simulink library "SLUGS_Library"  (Simulink 6.6)
values from neighbouring files (symbols this model uses):
  T = 0.01    [initGPS.m]    (also in mcuInit.m)
undefined symbols (not defined in the file or in its folder): apSampleTime, bankCommandLimit, daLimit, deLimit, DiscIntNeverNeededParam, drLimit, dtLimit, gaind, getWP, heightErrorLimit, mass, Ndelay, param, pitchCommandLimit, pitchErrorLimit, polesd, rollControlLimit, SampleT, Ts, u1, Xpoints, y1, yawDamperLimit, yo, Ypoints, zerosd, Zpoints
libraries: SLUGS_Library x51, simulink x32, dsPICdrivers x13, aerolibutil x2, aerolibconvert2 x1
(part 2 of 2)

== system SLUGS_Library/Singnal Routing & Conditioning/3D Filter ==
  In1 : Inport
  Demux : Demux  Outputs=3
  Filter1 : Subsystem  mask(DiscretizedZeroPole){Zeros=zval, Poles=pval, Gain=kval, AbsTol=auto, SampleTime=TSample, method=tustin, Wc=1}
      mask prompts: Zeros "Zeros (enter in s-main:)"; Poles "Poles (enter in s-domain:)"; Gain "Gain (enter in s-domain:)"; AbsTol "Absolute tolerance:"; SampleTime "Sample time:"; Wc "Critical Frequency (Hz):"
      mask help: Continuous mask uses c2d to transform parameters onto the Discrete Zero-Pole block inside.
      mask init: same as SLUGS_Library/Singnal Routing & Conditioning/Filter
      mask StyleString: edit,edit,edit,edit,edit,popup(zoh|foh|tustin|prewarp|matched),edit
      mask CallbackString: |||||hidecrit|
      mask Display:
      | droots(zeross,poless,gainss)
      | text( 0.5, 1.0, method, 'verticalAlignment','top')
  Filter2 : Subsystem  mask(DiscretizedZeroPole){Zeros=zval, Poles=pval, Gain=kval, AbsTol=auto, SampleTime=TSample, method=tustin, Wc=1}
      mask prompts: Zeros "Zeros (enter in s-main:)"; Poles "Poles (enter in s-domain:)"; Gain "Gain (enter in s-domain:)"; AbsTol "Absolute tolerance:"; SampleTime "Sample time:"; Wc "Critical Frequency (Hz):"
      mask help: Continuous mask uses c2d to transform parameters onto the Discrete Zero-Pole block inside.
      mask init: same as SLUGS_Library/Singnal Routing & Conditioning/Filter
      mask StyleString: edit,edit,edit,edit,edit,popup(zoh|foh|tustin|prewarp|matched),edit
      mask CallbackString: |||||hidecrit|
      mask Display:
      | droots(zeross,poless,gainss)
      | text( 0.5, 1.0, method, 'verticalAlignment','top')
  Filter3 : Subsystem  mask(DiscretizedZeroPole){Zeros=zval, Poles=pval, Gain=kval, AbsTol=auto, SampleTime=TSample, method=tustin, Wc=1}
      mask prompts: Zeros "Zeros (enter in s-main:)"; Poles "Poles (enter in s-domain:)"; Gain "Gain (enter in s-domain:)"; AbsTol "Absolute tolerance:"; SampleTime "Sample time:"; Wc "Critical Frequency (Hz):"
      mask help: Continuous mask uses c2d to transform parameters onto the Discrete Zero-Pole block inside.
      mask init: same as SLUGS_Library/Singnal Routing & Conditioning/Filter
      mask StyleString: edit,edit,edit,edit,edit,popup(zoh|foh|tustin|prewarp|matched),edit
      mask CallbackString: |||||hidecrit|
      mask Display:
      | droots(zeross,poless,gainss)
      | text( 0.5, 1.0, method, 'verticalAlignment','top')
  myMux Fun1 : Stateflow chart
  Out1 : Outport
  wires:
  Demux/1 -> Filter1/1(In1)
  Demux/2 -> Filter2/1(In1)
  Demux/3 -> Filter3/1(In1)
  Filter1/1(Out1) -> myMux Fun1/1(u1)
  Filter2/1(Out1) -> myMux Fun1/2(u2)
  Filter3/1(Out1) -> myMux Fun1/3(u3)
  In1/1 -> Demux/1
  myMux Fun1/1(y) -> Out1/1

== system SLUGS_Library/Singnal Routing & Conditioning/3D LowPass w/Initial Condition ==
  In : Inport
  Demux : Demux  Outputs=3
  Discrete Low Pass : Subsystem  mask{a=a, Yo=yo(1), Ts=T}
      mask prompts: a "Pole location (continuous)"; Yo "Initial condition"; Ts "Sample Time (seconds)"
      mask Display:
      | port_label('input',1,'U')
      | port_label('output',1,'Y')
      | text(0.35,0.85,'Tustin')
      | dpoly([a],[1 a],'s')
  Discrete Low Pass1 : Subsystem  mask{a=a, Yo=yo(2), Ts=T}
      mask prompts: a "Pole location (continuous)"; Yo "Initial condition"; Ts "Sample Time (seconds)"
      mask Display:
      | port_label('input',1,'U')
      | port_label('output',1,'Y')
      | text(0.35,0.85,'Tustin')
      | dpoly([a],[1 a],'s')
  Discrete Low Pass2 : Subsystem  mask{a=a, Yo=yo(3), Ts=T}
      mask prompts: a "Pole location (continuous)"; Yo "Initial condition"; Ts "Sample Time (seconds)"
      mask Display:
      | port_label('input',1,'U')
      | port_label('output',1,'Y')
      | text(0.35,0.85,'Tustin')
      | dpoly([a],[1 a],'s')
  myMux Fun1 : Stateflow chart
  Out1 : Outport
  wires:
  Discrete Low Pass2/1(Y) -> myMux Fun1/3(u3)
  Discrete Low Pass1/1(Y) -> myMux Fun1/2(u2)
  Discrete Low Pass/1(Y) -> myMux Fun1/1(u1)
  myMux Fun1/1(y) -> Out1/1
  Demux/1 -> Discrete Low Pass/1(U)
  Demux/2 -> Discrete Low Pass1/1(U)
  Demux/3 -> Discrete Low Pass2/1(U)
  In/1 -> Demux/1

== system SLUGS_Library/Singnal Routing & Conditioning/Discrete Low Pass w/initial condition ==
  U : Inport
  Gain : Gain  Orientation=left  Gain=(2-a*Ts)  SampleTime=Ts
  Gain1 : Gain  Gain=1/(2+a*Ts)  SampleTime=Ts
  Gain2 : Gain  Gain=a*Ts  SampleTime=Ts
  Sum : Sum  Inputs=++|
  Sum1 : Sum  Inputs=|++
  Unit Delay : UnitDelay  X0=Yo  SampleTime=Ts
  Unit Delay1 : UnitDelay  X0=Yo  SampleTime=Ts
  Y : Outport
  wires:
  Gain/1 -> Sum1/2
  Sum1/1 -> Gain1/1
  Gain2/1 -> Sum1/1
  Gain1/1 -> Y/1, Unit Delay/1  "Y_k"
  Sum/1 -> Gain2/1
  Unit Delay1/1 -> Sum/2  "U_k-1"
  U/1 -> Sum/1, Unit Delay1/1  "U_k"
  Unit Delay/1 -> Gain/1  "Y_k-1"

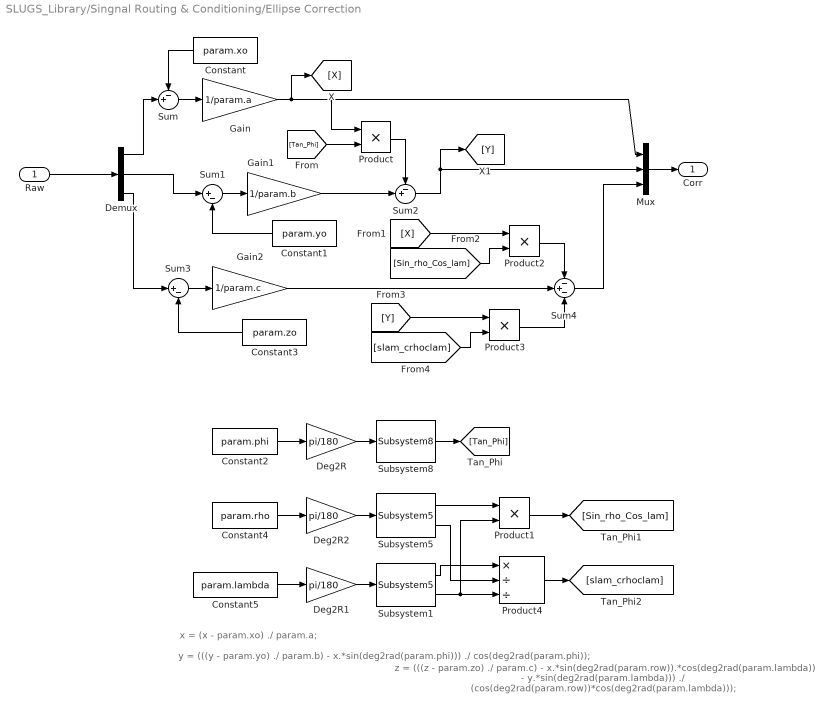
== system SLUGS_Library/Singnal Routing & Conditioning/Ellipse Correction ==
  note: z = (((z - param.zo) ./ param.c) - x.*sin(deg2rad(param.row)).*cos(deg2rad(param.lambda)) - y.*sin(deg2rad(param.lambda))) ./ (cos(deg2rad(param.row))*cos(deg2rad(param.lambda)));
  note: y = (((y - param.yo) ./ param.b) - x.*sin(deg2rad(param.phi))) ./ cos(deg2rad(param.phi));
  note: x = (x - param.xo) ./ param.a;
  Raw : Inport
  Constant : Constant  Orientation=left  Value=param.xo
  Constant1 : Constant  Orientation=left  Value=param.yo
  Constant2 : Constant  Value=param.phi  OutDataTypeMode=single
  Constant3 : Constant  Orientation=left  Value=param.zo
  Constant4 : Constant  Value=param.rho  OutDataTypeMode=single
  Constant5 : Constant  Value=param.lambda  OutDataTypeMode=single
  Deg2R : Gain  Gain=pi/180  SaturateOnIntegerOverflow=on
  Deg2R1 : Gain  Gain=pi/180  SaturateOnIntegerOverflow=on
  Deg2R2 : Gain  Gain=pi/180  SaturateOnIntegerOverflow=on
  Demux : Demux  Outputs=3
  Gain : Gain  Gain=1/param.a
  Gain1 : Gain  Gain=1/param.b
  Gain2 : Gain  Gain=1/param.c
  Mux : Mux  Inputs=3
  Product{,1..3} (4 alike) : Product  RndMeth=Zero
  Product4 : Product  Inputs=*//  RndMeth=Zero
  Subsystem1 : SLUGS_Library/Subsystem5  SystemSampleTime=-1
  Subsystem5 : SLUGS_Library/Subsystem5  SystemSampleTime=-1
  Subsystem8 : SLUGS_Library/Subsystem8  SystemSampleTime=-1
  Sum : Sum  Inputs=-+|
  Sum1 : Sum  Inputs=|+-
  Sum2 : Sum  Inputs=-+|
  Sum3 : Sum  Inputs=|+-
  Sum4 : Sum  Inputs=-+-
  Corr : Outport
  wires:
  Sum4/1 -> Mux/3
  Product4/1 -> [slam_crhoclam]
  Subsystem5/2 -> Product4/2
  Subsystem1/1 -> Product4/1
  Product3/1 -> Sum4/3
  [slam_crhoclam] -> Product3/2
  [Y] -> Product3/1
  Product2/1 -> Sum4/1
  [Sin_rho_Cos_lam] -> Product2/2
  [X] -> Product2/1
  Product1/1 -> [Sin_rho_Cos_lam]
  Subsystem1/2 -> Product4/3, Product1/2
  Subsystem5/1 -> Product1/1
  Deg2R1/1 -> Subsystem1/1
  Constant5/1 -> Deg2R1/1
  Deg2R2/1 -> Subsystem5/1
  Constant4/1 -> Deg2R2/1
  Demux/3 -> Sum3/1
  Gain2/1 -> Sum4/2
  Constant3/1 -> Sum3/2
  Sum3/1 -> Gain2/1
  Sum2/1 -> [Y], Mux/2
  Product/1 -> Sum2/1
  Gain1/1 -> Sum2/2
  [Tan_Phi] -> Product/2
  Subsystem8/1 -> [Tan_Phi]
  Deg2R/1 -> Subsystem8/1
  Constant2/1 -> Deg2R/1
  Demux/2 -> Sum1/1
  Constant1/1 -> Sum1/2
  Mux/1 -> Corr/1
  Sum1/1 -> Gain1/1
  Gain/1 -> Product/1, Mux/1, [X]
  Sum/1 -> Gain/1
  Constant/1 -> Sum/1
  Demux/1 -> Sum/2
  Raw/1 -> Demux/1

== system SLUGS_Library/Singnal Routing & Conditioning/Filter ==
  In1 : Inport
  Discrete Zero-Pole : DiscreteZeroPole  Zeros=zerosd  Poles=polesd  Gain=gaind  SampleTime=SampleTime
  Out1 : Outport
  wires:
  Discrete Zero-Pole/1 -> Out1/1
  In1/1 -> Discrete Zero-Pole/1

== system SLUGS_Library/Singnal Routing & Conditioning/Zero Limit ==
  In : Inport
  Compare To Zero : simulink/Logic and Bit Operations/Compare To Zero  SystemSampleTime=-1  relop=<  LogicOutDataTypeMode=uint8  ZeroCross=off
  Constant : Constant  Value=0
  Switch : Switch  Threshold=0.1
  Zero Limit Out : Outport
  wires:
  Compare To Zero/1 -> Switch/2
  Constant/1 -> Switch/1
  In/1 -> Compare To Zero/1, Switch/3
  Switch/1 -> Zero Limit Out/1

== system SLUGS_Library/Control Blocks/PD Controller  Internal Derivative/Low_passed Time Derivative ==
  f(t) : Inport
  Add : Sum  OutScaling=2^-10
  Constant : Constant  Value=NDelay*TSample  OutDataTypeMode=single
  Divide : Product  Inputs=*/  OutScaling=2^-10
  Integer Delay : simulink/Discrete/Integer Delay  vinit=0.0  samptime=TSample  NumDelays=NDelay
  f_dot(t) : Outport
  wires:
  Divide/1 -> f_dot(t)/1
  Constant/1 -> Divide/2
  Integer Delay/1 -> Add/2
  f(t)/1 -> Integer Delay/1, Add/1
  Add/1 -> Divide/1

== system SLUGS_Library/Control Blocks/PID Controller/Low_passed Time Derivative ==
  f(t) : Inport
  Add : Sum  OutScaling=2^-10
  Constant : Constant  Value=NDelay*TSample  OutDataTypeMode=single
  Divide : Product  Inputs=*/  OutDataTypeMode=single  OutScaling=2^-10
  Integer Delay : simulink/Discrete/Integer Delay  vinit=0.0  samptime=TSample  NumDelays=NDelay
  f_dot(t) : Outport
  wires:
  Add/1 -> Divide/1
  f(t)/1 -> Add/1, Integer Delay/1
  Integer Delay/1 -> Add/2
  Constant/1 -> Divide/2
  Divide/1 -> f_dot(t)/1

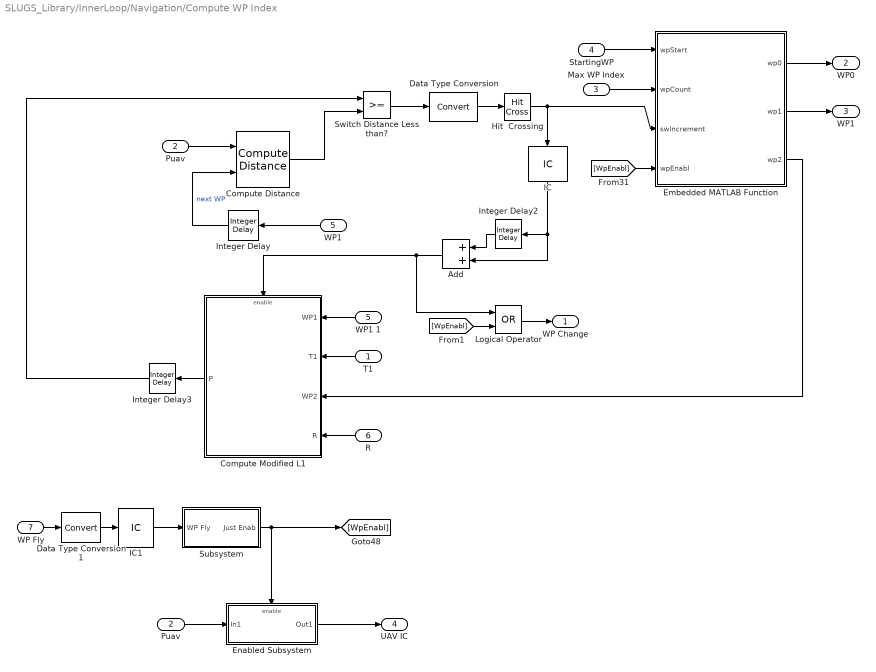
== system SLUGS_Library/InnerLoop/Navigation/Compute WP Index ==
  T1 : Inport  Orientation=left
  Puav : Inport  Port=2
  Max WP Index : Inport  Port=3
  StartingWP : Inport  Port=4
  "WP1 " : Inport  Orientation=left  Port=5
  R : Inport  Orientation=left  Port=6
  WP Fly : Inport  Port=7
  Add : Sum  Orientation=left  Inputs=2  OutScaling=2^-10
  Compute Distance : SLUGS_Library/Navigation/Compute Distance  SystemSampleTime=-1
  Compute Modified L1 : Subsystem  Orientation=left
  Data Type Conversion : DataTypeConversion  OutDataTypeMode=double  SampleTime=apSampleTime
  Data Type Conversion1 : DataTypeConversion  OutDataTypeMode=double  SampleTime=apSampleTime
  Embedded MATLAB Function : Stateflow chart
  Enabled Subsystem : Subsystem  TreatAsAtomicUnit=on
  Hit  Crossing : HitCross  HitCrossingOffset=0.9  HitCrossingDirection=rising  SampleTime=apSampleTime
  IC : InitialCondition  Orientation=down
  IC1 : InitialCondition  Value=0
  Integer Delay : simulink/Discrete/Integer Delay  Orientation=left  vinit=0.0  samptime=-1  NumDelays=1
  Integer Delay2 : simulink/Discrete/Integer Delay  Orientation=left  vinit=0  samptime=-1  NumDelays=1
  Integer Delay3 : simulink/Discrete/Integer Delay  Orientation=left  vinit=150  samptime=-1  NumDelays=1
  Logical Operator : Logic  Operator=OR  AllPortsSameDT=off  OutDataTypeMode=Boolean
  "Puav " : InportShadow  Port=2  LatchByCopyingInsideSignal=off
  Subsystem : Subsystem
  Switch Distance Less than? : RelationalOperator  LogicOutDataTypeMode=Boolean  LogicDataType=double()  SampleTime=apSampleTime
  WP1 1 : InportShadow  Orientation=left  Port=5  LatchByCopyingInsideSignal=off
  WP Change : Outport
  WP0 : Outport  Port=2
  WP1 : Outport  Port=3
  UAV IC : Outport  Port=4
  wires:
  [WpEnabl] -> Logical Operator/2
  Logical Operator/1 -> WP Change/1
  [WpEnabl] -> Embedded MATLAB Function/4(wpEnabl)
  IC1/1 -> Subsystem/1(WP Fly)
  Enabled Subsystem/1(Out1) -> UAV IC/1
  "Puav "/1 -> Enabled Subsystem/1(In1)
  Subsystem/1(Just Enab) -> [WpEnabl], Enabled Subsystem/Enable
  WP Fly/1 -> Data Type Conversion1/1
  R/1 -> Compute Modified L1/4(R)
  Integer Delay3/1 -> Switch Distance Less than?/1
  Compute Modified L1/1(P) -> Integer Delay3/1
  IC/1 -> Integer Delay2/1, Add/2
  Add/1 -> Logical Operator/1, Compute Modified L1/Enable
  Integer Delay2/1 -> Add/1
  T1/1 -> Compute Modified L1/2(T1)
  WP1 1/1 -> Compute Modified L1/1(WP1)
  Embedded MATLAB Function/3(wp2) -> Compute Modified L1/3(WP2)
  Data Type Conversion/1 -> Hit  Crossing/1
  Hit  Crossing/1 -> IC/1, Embedded MATLAB Function/3(swIncrement)
  "WP1 "/1 -> Integer Delay/1
  Compute Distance/1 -> Switch Distance Less than?/2
  Max WP Index/1 -> Embedded MATLAB Function/2(wpCount)
  Switch Distance Less than?/1 -> Data Type Conversion/1
  StartingWP/1 -> Embedded MATLAB Function/1(wpStart)
  Embedded MATLAB Function/1(wp0) -> WP0/1
  Embedded MATLAB Function/2(wp1) -> WP1/1
  Puav/1 -> Compute Distance/1
  Integer Delay/1 -> Compute Distance/2  "next WP"
  Data Type Conversion1/1 -> IC1/1

== system SLUGS_Library/InnerLoop/Navigation/Get Wps Compute Frenet ==
  WP Idx 0 : Inport
  WP Idx 1 : Inport  Port=2
  UAV IC : Inport  Port=3
  Enable : EnablePort
  Compute Frenet : SLUGS_Library/Navigation/Compute Frenet  SystemSampleTime=-1
  Switch : Switch  Criteria=u2 > Threshold  Threshold=0.3
  get WP Coord from Index : SLUGS_Library/Navigation/get WP Coord from Index  SystemSampleTime=-1
  "get WP Coord from Index " : SLUGS_Library/Navigation/get WP Coord from Index  SystemSampleTime=-1
  T : Outport
  N : Outport  Port=2
  WP 1 : Outport  Port=3
  wires:
  WP Idx 0/1 -> get WP Coord from Index/1, Switch/2
  Compute Frenet/1 -> T/1
  Compute Frenet/2 -> N/1
  WP Idx 1/1 -> "get WP Coord from Index "/1
  "get WP Coord from Index "/1 -> Compute Frenet/2, WP 1/1
  Switch/1 -> Compute Frenet/1
  get WP Coord from Index/1 -> Switch/1
  UAV IC/1 -> Switch/3

== system SLUGS_Library/Navigation/Compute WP Index/Compute Modified L1 ==
  WP1 : Inport  Orientation=left
  T1 : Inport  Port=2
  WP2 : Inport  Orientation=left  Port=3
  R : Inport  Port=4
  Enable : EnablePort  ShowOutputPort=on
  Compute T  in Frenet : Subsystem  Orientation=left  AncestorBlock=SLUGS_Library/Navigation/Compute Frenet
  Get Circles : Subsystem
  Integer Delay1 : simulink/Discrete/Integer Delay  vinit=0.0  samptime=-1  NumDelays=1
  Integer Delay2 : simulink/Discrete/Integer Delay  Orientation=left  vinit=0.0  samptime=-1  NumDelays=1
  To Workspace : ToWorkspace  VariableName=wpChange  SampleTime=-1  SaveFormat=Structure
  WP1_1 : InportShadow  Port=1  LatchByCopyingInsideSignal=off
  get WP Coord from Index : SLUGS_Library/Navigation/get WP Coord from Index  Orientation=left  SystemSampleTime=-1
  P : Outport
  wires:
  get WP Coord from Index/1 -> Integer Delay2/1
  Integer Delay2/1 -> Compute T  in Frenet/2(Pos 2)
  Compute T  in Frenet/1(T) -> Get Circles/2(T2)
  WP1/1 -> Compute T  in Frenet/1(Pos 1)
  WP2/1 -> get WP Coord from Index/1
  T1/1 -> Integer Delay1/1
  Get Circles/1(P) -> P/1
  WP1_1/1 -> Get Circles/3("Wp_to ")
  Integer Delay1/1 -> Get Circles/1(T1)
  Enable/1 -> To Workspace/1
  R/1 -> Get Circles/4(R)

== system SLUGS_Library/Navigation/Compute WP Index/Enabled Subsystem ==
  In1 : Inport
  Enable : EnablePort
  Out1 : Outport
  wires:
  In1/1 -> Out1/1

== system SLUGS_Library/Navigation/Compute WP Index/Subsystem ==
  WP Fly : Inport
  Add1 : Sum  Inputs=2  OutScaling=2^-10
  Hit  Crossing1 : HitCross  HitCrossingOffset=0.3  HitCrossingDirection=rising  SampleTime=apSampleTime
  Integer Delay1 : simulink/Discrete/Integer Delay  vinit=0  samptime=-1  NumDelays=1
  Just Enab : Outport
  wires:
  Integer Delay1/1 -> Add1/1
  Hit  Crossing1/1 -> Add1/2, Integer Delay1/1
  Add1/1 -> Just Enab/1
  WP Fly/1 -> Hit  Crossing1/1

== system SLUGS_Library/Navigation/Park, Deyst & How Lat Accel Cmd/Compute Eta ==
  Vxyz : Inport
  L1_vec : Inport  Port=2
  3x3 Cross Product : aerolibutil/3x3 Cross Product  SystemSampleTime=-1
  Divide5 : Product  Inputs=*//  OutScaling=2^-10
  Norm : SLUGS_Library/Navigation/Norm  SystemSampleTime=-1
  "Norm " : SLUGS_Library/Navigation/Norm  SystemSampleTime=-1
  Selector : Selector  IndexOptions=Index vector (dialog)  Indices=[3]  OutputSizes=1  InputPortWidth=3
  Subsystem6 : SLUGS_Library/Subsystem6  SystemSampleTime=-1
  To Workspace : ToWorkspace  VariableName=L1  SampleTime=-1  SaveFormat=Array
  To Workspace1 : ToWorkspace  VariableName=Vned  SampleTime=-1  SaveFormat=Array
  To Workspace2 : ToWorkspace  VariableName=eta  SampleTime=-1  SaveFormat=Array
  negprotect : Stateflow chart
  negprotect1 : Stateflow chart
  Eta : Outport
  wires:
  Subsystem6/1 -> To Workspace2/1, Eta/1
  Selector/1 -> Subsystem6/1
  Vxyz/1 -> "Norm "/1, To Workspace1/1, 3x3 Cross Product/1
  3x3 Cross Product/1 -> Divide5/1
  Norm/1 -> negprotect/1(val)
  "Norm "/1 -> negprotect1/1(val)
  Divide5/1 -> Selector/1
  L1_vec/1 -> Norm/1, 3x3 Cross Product/2, To Workspace/1
  negprotect1/1(zpVal) -> Divide5/3
  negprotect/1(zpVal) -> Divide5/2

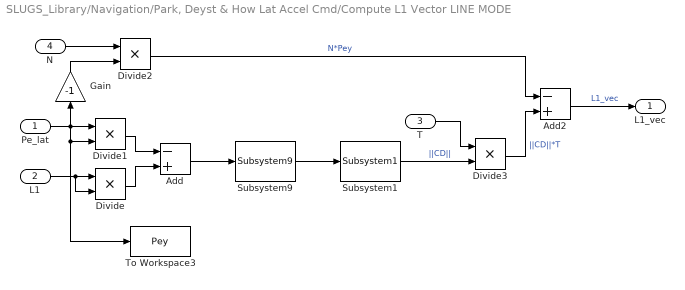
== system SLUGS_Library/Navigation/Park, Deyst & How Lat Accel Cmd/Compute L1 Vector LINE MODE ==
  Pe_lat : Inport
  L1 : Inport  Port=2
  T : Inport  Port=3
  N : Inport  Port=4
  Add : Sum  Inputs=-+  OutScaling=2^-10
  Add2 : Sum  Inputs=-+  OutScaling=2^-10
  Divide{,1..3} (4 alike) : Product  OutScaling=2^-10
  Gain : Gain  Orientation=up  Gain=-1
  Subsystem1 : SLUGS_Library/Subsystem1  SystemSampleTime=-1
  Subsystem9 : SLUGS_Library/Subsystem9  SystemSampleTime=-1
  To Workspace3 : ToWorkspace  VariableName=Pey  SampleTime=-1  SaveFormat=Array
  L1_vec : Outport
  wires:
  Subsystem9/1 -> Subsystem1/1
  Add2/1 -> L1_vec/1  "L1_vec"
  Gain/1 -> Divide2/2
  L1/1 -> Divide/1, Divide/2
  Pe_lat/1 -> Gain/1, To Workspace3/1, Divide1/2, Divide1/1
  Divide1/1 -> Add/1
  Divide/1 -> Add/2
  Add/1 -> Subsystem9/1
  Subsystem1/1 -> Divide3/2  "||CD||"
  Divide2/1 -> Add2/1  "N*Pey"
  N/1 -> Divide2/1
  T/1 -> Divide3/1
  Divide3/1 -> Add2/2  "||CD||*T"

== system SLUGS_Library/Navigation/Park, Deyst & How Lat Accel Cmd/Park's Lateral Accel Command ==
  Vxyz : Inport
  L1 : Inport  Port=2
  eta : Inport  Port=3
  Constant : Constant  Value=2
  Norm : SLUGS_Library/Navigation/Norm  SystemSampleTime=-1
  Product : Product  Inputs=***/*  RndMeth=Zero
  Subsystem7 : SLUGS_Library/Subsystem7  SystemSampleTime=-1
  a_s_c : Outport
  wires:
  eta/1 -> Subsystem7/1
  Vxyz/1 -> Norm/1
  Norm/1 -> Product/1, Product/2
  Constant/1 -> Product/3
  L1/1 -> Product/4
  Subsystem7/1 -> Product/5
  Product/1 -> a_s_c/1

== system SLUGS_Library/Singnal Routing & Conditioning/3D Filter/Filter1 ==
  In1 : Inport
  Discrete Zero-Pole : DiscreteZeroPole  Zeros=zerosd  Poles=polesd  Gain=gaind  SampleTime=SampleTime
  Out1 : Outport
  wires:
  In1/1 -> Discrete Zero-Pole/1
  Discrete Zero-Pole/1 -> Out1/1

== system SLUGS_Library/Singnal Routing & Conditioning/3D Filter/Filter2 ==
  In1 : Inport
  Discrete Zero-Pole : DiscreteZeroPole  Zeros=zerosd  Poles=polesd  Gain=gaind  SampleTime=SampleTime
  Out1 : Outport
  wires:
  Discrete Zero-Pole/1 -> Out1/1
  In1/1 -> Discrete Zero-Pole/1

== system SLUGS_Library/Singnal Routing & Conditioning/3D Filter/Filter3 ==
  In1 : Inport
  Discrete Zero-Pole : DiscreteZeroPole  Zeros=zerosd  Poles=polesd  Gain=gaind  SampleTime=SampleTime
  Out1 : Outport
  wires:
  In1/1 -> Discrete Zero-Pole/1
  Discrete Zero-Pole/1 -> Out1/1

== system SLUGS_Library/Singnal Routing & Conditioning/3D LowPass w/Initial Condition/Discrete Low Pass ==
  U : Inport
  Gain : Gain  Orientation=left  Gain=(2-a*Ts)  SampleTime=Ts
  Gain1 : Gain  Gain=1/(2+a*Ts)  SampleTime=Ts
  Gain2 : Gain  Gain=a*Ts  SampleTime=Ts
  Sum : Sum  Inputs=++|
  Sum1 : Sum  Inputs=|++
  Unit Delay : UnitDelay  X0=Yo  SampleTime=Ts
  Unit Delay1 : UnitDelay  X0=Yo  SampleTime=Ts
  Y : Outport
  wires:
  Gain/1 -> Sum1/2
  Sum1/1 -> Gain1/1
  Gain2/1 -> Sum1/1
  Gain1/1 -> Y/1, Unit Delay/1  "Y_k"
  Sum/1 -> Gain2/1
  Unit Delay1/1 -> Sum/2  "U_k-1"
  U/1 -> Sum/1, Unit Delay1/1  "U_k"
  Unit Delay/1 -> Gain/1  "Y_k-1"

== system SLUGS_Library/Singnal Routing & Conditioning/3D LowPass w/Initial Condition/Discrete Low Pass1 ==
  U : Inport
  Gain : Gain  Orientation=left  Gain=(2-a*Ts)  SampleTime=Ts
  Gain1 : Gain  Gain=1/(2+a*Ts)  SampleTime=Ts
  Gain2 : Gain  Gain=a*Ts  SampleTime=Ts
  Sum : Sum  Inputs=++|
  Sum1 : Sum  Inputs=|++
  Unit Delay : UnitDelay  X0=Yo  SampleTime=Ts
  Unit Delay1 : UnitDelay  X0=Yo  SampleTime=Ts
  Y : Outport
  wires:
  Gain/1 -> Sum1/2
  Sum1/1 -> Gain1/1
  Gain2/1 -> Sum1/1
  Gain1/1 -> Y/1, Unit Delay/1  "Y_k"
  Sum/1 -> Gain2/1
  Unit Delay1/1 -> Sum/2  "U_k-1"
  U/1 -> Sum/1, Unit Delay1/1  "U_k"
  Unit Delay/1 -> Gain/1  "Y_k-1"

== system SLUGS_Library/Singnal Routing & Conditioning/3D LowPass w/Initial Condition/Discrete Low Pass2 ==
  U : Inport
  Gain : Gain  Orientation=left  Gain=(2-a*Ts)  SampleTime=Ts
  Gain1 : Gain  Gain=1/(2+a*Ts)  SampleTime=Ts
  Gain2 : Gain  Gain=a*Ts  SampleTime=Ts
  Sum : Sum  Inputs=++|
  Sum1 : Sum  Inputs=|++
  Unit Delay : UnitDelay  X0=Yo  SampleTime=Ts
  Unit Delay1 : UnitDelay  X0=Yo  SampleTime=Ts
  Y : Outport
  wires:
  Gain/1 -> Sum1/2
  Sum1/1 -> Gain1/1
  Gain2/1 -> Sum1/1
  Gain1/1 -> Y/1, Unit Delay/1  "Y_k"
  Sum/1 -> Gain2/1
  Unit Delay1/1 -> Sum/2  "U_k-1"
  U/1 -> Sum/1, Unit Delay1/1  "U_k"
  Unit Delay/1 -> Gain/1  "Y_k-1"

== system SLUGS_Library/InnerLoop/Navigation/Compute WP Index/Compute Modified L1 ==
  WP1 : Inport  Orientation=left
  T1 : Inport  Port=2
  WP2 : Inport  Orientation=left  Port=3
  R : Inport  Port=4
  Enable : EnablePort  ShowOutputPort=on
  Compute T  in Frenet : Subsystem  Orientation=left  AncestorBlock=SLUGS_Library/Navigation/Compute Frenet
  Get Circles : Subsystem
  Integer Delay1 : simulink/Discrete/Integer Delay  vinit=0.0  samptime=-1  NumDelays=1
  Integer Delay2 : simulink/Discrete/Integer Delay  Orientation=left  vinit=0.0  samptime=-1  NumDelays=1
  To Workspace : ToWorkspace  VariableName=wpChange  SampleTime=-1  SaveFormat=Structure
  WP1_1 : InportShadow  Port=1  LatchByCopyingInsideSignal=off
  get WP Coord from Index : Subsystem  Orientation=left  AncestorBlock=SLUGS_Library/Navigation/get WP Coord from Index
  P : Outport
  wires:
  R/1 -> Get Circles/4(R)
  Enable/1 -> To Workspace/1
  Integer Delay1/1 -> Get Circles/1(T1)
  WP1_1/1 -> Get Circles/3("Wp_to ")
  Get Circles/1(P) -> P/1
  T1/1 -> Integer Delay1/1
  WP2/1 -> get WP Coord from Index/1(WP Idx)
  WP1/1 -> Compute T  in Frenet/1(Pos 1)
  Compute T  in Frenet/1(T) -> Get Circles/2(T2)
  Integer Delay2/1 -> Compute T  in Frenet/2(Pos 2)
  get WP Coord from Index/1(WP Coord) -> Integer Delay2/1

== system SLUGS_Library/InnerLoop/Navigation/Compute WP Index/Enabled Subsystem ==
  In1 : Inport
  Enable : EnablePort
  Out1 : Outport
  wires:
  In1/1 -> Out1/1

== system SLUGS_Library/InnerLoop/Navigation/Compute WP Index/Subsystem ==
  WP Fly : Inport
  Add1 : Sum  Inputs=2  OutScaling=2^-10
  Hit  Crossing1 : HitCross  HitCrossingOffset=0.3  HitCrossingDirection=rising  SampleTime=apSampleTime
  Integer Delay1 : simulink/Discrete/Integer Delay  vinit=0  samptime=-1  NumDelays=1
  Just Enab : Outport
  wires:
  WP Fly/1 -> Hit  Crossing1/1
  Add1/1 -> Just Enab/1
  Hit  Crossing1/1 -> Integer Delay1/1, Add1/2
  Integer Delay1/1 -> Add1/1

== system SLUGS_Library/Navigation/Compute WP Index/Compute Modified L1/Compute T  in Frenet ==
  Pos 1 : Inport
  Pos 2 : Inport  Port=2
  Add : Sum  Inputs=-+  OutScaling=2^-10
  Normalize Vector : SLUGS_Library/Navigation/Normalize Vector  SystemSampleTime=-1
  T : Outport
  wires:
  Normalize Vector/1 -> T/1
  Add/1 -> Normalize Vector/1
  Pos 2/1 -> Add/2
  Pos 1/1 -> Add/1

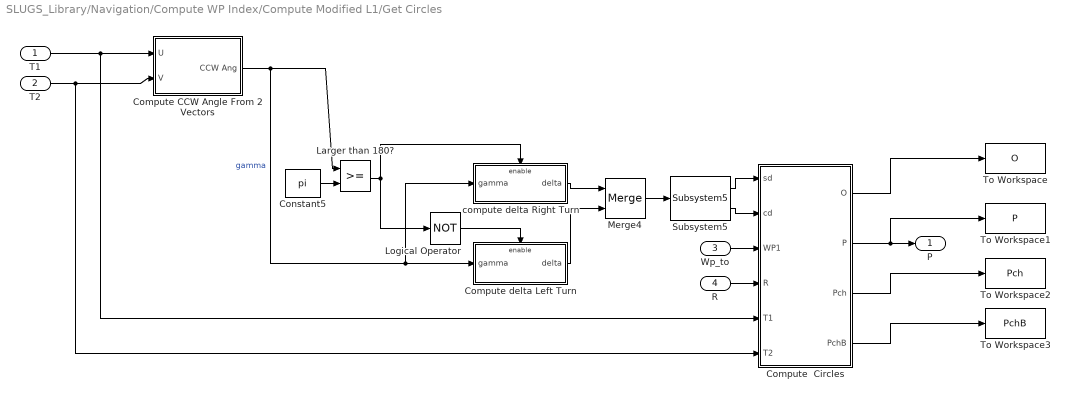
== system SLUGS_Library/Navigation/Compute WP Index/Compute Modified L1/Get Circles ==
  T1 : Inport
  T2 : Inport  Port=2
  "Wp_to " : Inport  Port=3
  R : Inport  Port=4
  Compute  Circles : Stateflow chart
  Compute CCW Angle From 2 Vectors : Subsystem
  Compute delta Left Turn : Subsystem
  Constant5 : Constant  Value=pi
  Larger than 180? : RelationalOperator  LogicOutDataTypeMode=Boolean  LogicDataType=double()
  Logical Operator : Logic  Operator=NOT  AllPortsSameDT=off  OutDataTypeMode=Boolean
  Merge4 : Merge
  Subsystem5 : SLUGS_Library/Subsystem5  SystemSampleTime=-1
  To Workspace : ToWorkspace  VariableName=O  SampleTime=-1  SaveFormat=Structure
  To Workspace1 : ToWorkspace  VariableName=P  SampleTime=-1  SaveFormat=Structure
  To Workspace2 : ToWorkspace  VariableName=Pch  SampleTime=-1  SaveFormat=Structure
  To Workspace3 : ToWorkspace  VariableName=PchB  SampleTime=-1  SaveFormat=Structure
  compute delta Right Turn : Subsystem
  P : Outport
  wires:
  T1/1 -> Compute  Circles/5(T1), Compute CCW Angle From 2 Vectors/1(U)
  Compute CCW Angle From 2 Vectors/1(CCW Ang) -> Compute delta Left Turn/1(gamma), compute delta Right Turn/1(gamma), Larger than 180?/1  "gamma"
  T2/1 -> Compute  Circles/6(T2), Compute CCW Angle From 2 Vectors/2(V)
  Merge4/1 -> Subsystem5/1
  compute delta Right Turn/1(delta) -> Merge4/1
  Compute delta Left Turn/1(delta) -> Merge4/2
  R/1 -> Compute  Circles/4(R)
  "Wp_to "/1 -> Compute  Circles/3(WP1)
  Compute  Circles/1(O) -> To Workspace/1
  Compute  Circles/2(P) -> P/1, To Workspace1/1
  Compute  Circles/3(Pch) -> To Workspace2/1
  Compute  Circles/4(PchB) -> To Workspace3/1
  Constant5/1 -> Larger than 180?/2
  Larger than 180?/1 -> compute delta Right Turn/Enable, Logical Operator/1
  Logical Operator/1 -> Compute delta Left Turn/Enable
  Subsystem5/1 -> Compute  Circles/1(sd)
  Subsystem5/2 -> Compute  Circles/2(cd)

== system SLUGS_Library/InnerLoop/Navigation/Compute WP Index/Compute Modified L1/Compute T  in Frenet ==
  Pos 1 : Inport
  Pos 2 : Inport  Port=2
  Add : Sum  Inputs=-+  OutScaling=2^-10
  Normalize Vector : SLUGS_Library/Navigation/Normalize Vector  SystemSampleTime=-1
  T : Outport
  wires:
  Pos 1/1 -> Add/1
  Pos 2/1 -> Add/2
  Add/1 -> Normalize Vector/1
  Normalize Vector/1 -> T/1

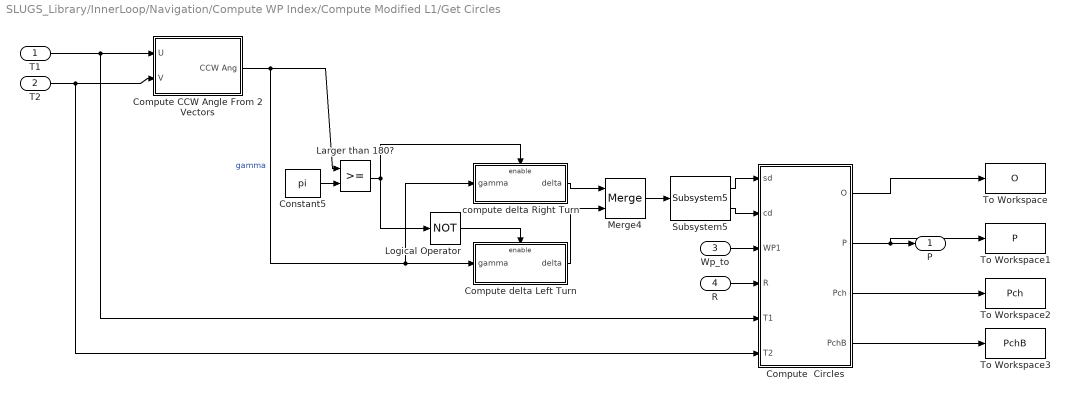
== system SLUGS_Library/InnerLoop/Navigation/Compute WP Index/Compute Modified L1/Get Circles ==
  T1 : Inport
  T2 : Inport  Port=2
  "Wp_to " : Inport  Port=3
  R : Inport  Port=4
  Compute  Circles : Stateflow chart
  Compute CCW Angle From 2 Vectors : Subsystem
  Compute delta Left Turn : Subsystem
  Constant5 : Constant  Value=pi  OutDataTypeMode=single
  Larger than 180? : RelationalOperator  LogicOutDataTypeMode=Boolean  LogicDataType=double()
  Logical Operator : Logic  Operator=NOT  AllPortsSameDT=off  OutDataTypeMode=Boolean
  Merge4 : Merge
  Subsystem5 : SLUGS_Library/Subsystem5  SystemSampleTime=-1
  To Workspace : ToWorkspace  VariableName=O  SampleTime=-1  SaveFormat=Structure
  To Workspace1 : ToWorkspace  VariableName=P  SampleTime=-1  SaveFormat=Structure
  To Workspace2 : ToWorkspace  VariableName=Pch  SampleTime=-1  SaveFormat=Structure
  To Workspace3 : ToWorkspace  VariableName=PchB  SampleTime=-1  SaveFormat=Structure
  compute delta Right Turn : Subsystem
  P : Outport
  wires:
  Subsystem5/2 -> Compute  Circles/2(cd)
  Subsystem5/1 -> Compute  Circles/1(sd)
  Logical Operator/1 -> Compute delta Left Turn/Enable
  Larger than 180?/1 -> Logical Operator/1, compute delta Right Turn/Enable
  Constant5/1 -> Larger than 180?/2
  Compute  Circles/4(PchB) -> To Workspace3/1
  Compute  Circles/3(Pch) -> To Workspace2/1
  Compute  Circles/2(P) -> To Workspace1/1, P/1
  Compute  Circles/1(O) -> To Workspace/1
  "Wp_to "/1 -> Compute  Circles/3(WP1)
  R/1 -> Compute  Circles/4(R)
  Compute delta Left Turn/1(delta) -> Merge4/2
  compute delta Right Turn/1(delta) -> Merge4/1
  Merge4/1 -> Subsystem5/1
  T2/1 -> Compute CCW Angle From 2 Vectors/2(V), Compute  Circles/6(T2)
  Compute CCW Angle From 2 Vectors/1(CCW Ang) -> Larger than 180?/1, compute delta Right Turn/1(gamma), Compute delta Left Turn/1(gamma)  "gamma"
  T1/1 -> Compute CCW Angle From 2 Vectors/1(U), Compute  Circles/5(T1)

== system SLUGS_Library/InnerLoop/Navigation/Compute WP Index/Compute Modified L1/get WP Coord from Index ==
  WP Idx : Inport
  C Function Call : dsPICdrivers/OTHERS/C Function Call  Tag=dsPIC_dsPIC_CFunctionCall  fctName='getWP'  INPUT_SIZE=1  INPUT1=uint8  INPUT2=--  INPUT3=--  OUTPUT_SIZE=3  OUTPUT1=real32  SampleTime=-1  InputType=[ 2 ]  OutputType=[ 7 ]  FctDeclaration=extern void getWP(uint8_T u1,real32_T* y1);  FctCall=getWP(%u1, *%y1);  OrderingInOutPopup=None
  Data Type Conversion : DataTypeConversion  OutDataTypeMode=double
  Data Type Conversion1 : DataTypeConversion  OutDataTypeMode=single
  Environment Controller : simulink/Signal Routing/Environment Controller  SystemSampleTime=-1
  MATLAB Fcn : MATLABFcn  MATLABFcn=Xpoints(u(1))  OutputDimensions=1  OutputSignalType=real
  MATLAB Fcn1 : MATLABFcn  MATLABFcn=Ypoints(u(1))  OutputDimensions=1
  MATLAB Fcn2 : MATLABFcn  MATLABFcn=Zpoints(u(1))  OutputDimensions=1
  Mux : Mux  Inputs=3
  WP Coord : Outport
  wires:
  C Function Call/1 -> Environment Controller/2
  Environment Controller/1 -> WP Coord/1
  Mux/1 -> Data Type Conversion1/1
  WP Idx/1 -> C Function Call/1, Data Type Conversion/1
  MATLAB Fcn2/1 -> Mux/3
  MATLAB Fcn1/1 -> Mux/2
  MATLAB Fcn/1 -> Mux/1
  Data Type Conversion/1 -> MATLAB Fcn1/1, MATLAB Fcn/1, MATLAB Fcn2/1
  Data Type Conversion1/1 -> Environment Controller/1

== system SLUGS_Library/Navigation/Compute WP Index/Compute Modified L1/Get Circles/Compute CCW Angle From 2 Vectors ==
  U : Inport
  V : Inport  Port=2
  Add : Sum  Inputs=+-  OutScaling=2^-10
  Embedded MATLAB Function1 : Stateflow chart
  Selector : Selector  IndexOptions=Index vector (dialog)  Indices=[1]  OutputSizes=1  InputPortWidth=3
  Selector1 : Selector  IndexOptions=Index vector (dialog)  Indices=[1]  OutputSizes=1  InputPortWidth=3
  Selector2 : Selector  IndexOptions=Index vector (dialog)  Indices=[2]  OutputSizes=1  InputPortWidth=3
  Selector3 : Selector  IndexOptions=Index vector (dialog)  Indices=[2]  OutputSizes=1  InputPortWidth=3
  Subsystem1 : SLUGS_Library/Subsystem4  SystemSampleTime=-1
  Subsystem4 : SLUGS_Library/Subsystem4  SystemSampleTime=-1
  CCW Ang : Outport
  wires:
  Selector3/1 -> Subsystem4/1
  Selector/1 -> Subsystem4/2
  Selector2/1 -> Subsystem1/1
  Selector1/1 -> Subsystem1/2
  Subsystem4/1 -> Add/1
  Subsystem1/1 -> Add/2
  Add/1 -> Embedded MATLAB Function1/1(rawAngle)
  U/1 -> Selector3/1, Selector/1
  V/1 -> Selector2/1, Selector1/1
  Embedded MATLAB Function1/1(angle) -> CCW Ang/1

== system SLUGS_Library/Navigation/Compute WP Index/Compute Modified L1/Get Circles/Compute delta Left Turn ==
  gamma : Inport
  Enable : EnablePort
  Add : Sum  Inputs=+-  OutScaling=2^-10
  Constant1 : Constant  Value=2
  Constant5 : Constant  Value=pi
  Divide : Product  Inputs=*/  OutScaling=2^-10
  Gain : Gain  Gain=-1
  delta : Outport
  wires:
  Constant1/1 -> Divide/2
  Divide/1 -> Gain/1
  Constant5/1 -> Add/1
  gamma/1 -> Add/2
  Add/1 -> Divide/1
  Gain/1 -> delta/1

== system SLUGS_Library/Navigation/Compute WP Index/Compute Modified L1/Get Circles/compute delta Right Turn ==
  gamma : Inport
  Enable : EnablePort
  Add : Sum  Inputs=-+  OutScaling=2^-10
  Constant1 : Constant  Value=2
  Constant5 : Constant  Value=pi
  Divide : Product  Inputs=*/  OutScaling=2^-10
  delta : Outport
  wires:
  Constant5/1 -> Add/1
  Add/1 -> Divide/1
  Constant1/1 -> Divide/2
  gamma/1 -> Add/2
  Divide/1 -> delta/1  "delta"

== system SLUGS_Library/InnerLoop/Navigation/Compute WP Index/Compute Modified L1/Get Circles/Compute CCW Angle From 2 Vectors ==
  U : Inport
  V : Inport  Port=2
  Add : Sum  Inputs=+-  OutScaling=2^-10
  Embedded MATLAB Function1 : Stateflow chart
  Selector : Selector  IndexOptions=Index vector (dialog)  Indices=[1]  OutputSizes=1  InputPortWidth=3
  Selector1 : Selector  IndexOptions=Index vector (dialog)  Indices=[1]  OutputSizes=1  InputPortWidth=3
  Selector2 : Selector  IndexOptions=Index vector (dialog)  Indices=[2]  OutputSizes=1  InputPortWidth=3
  Selector3 : Selector  IndexOptions=Index vector (dialog)  Indices=[2]  OutputSizes=1  InputPortWidth=3
  Subsystem1 : SLUGS_Library/Subsystem4  SystemSampleTime=-1
  Subsystem4 : SLUGS_Library/Subsystem4  SystemSampleTime=-1
  CCW Ang : Outport
  wires:
  Embedded MATLAB Function1/1(angle) -> CCW Ang/1
  V/1 -> Selector1/1, Selector2/1
  U/1 -> Selector/1, Selector3/1
  Add/1 -> Embedded MATLAB Function1/1(rawAngle)
  Subsystem1/1 -> Add/2
  Subsystem4/1 -> Add/1
  Selector1/1 -> Subsystem1/2
  Selector2/1 -> Subsystem1/1
  Selector/1 -> Subsystem4/2
  Selector3/1 -> Subsystem4/1

== system SLUGS_Library/InnerLoop/Navigation/Compute WP Index/Compute Modified L1/Get Circles/Compute delta Left Turn ==
  gamma : Inport
  Enable : EnablePort
  Add : Sum  Inputs=+-  OutDataTypeMode=single  OutScaling=2^-10
  Constant1 : Constant  Value=2  OutDataTypeMode=single
  Constant5 : Constant  Value=pi  OutDataTypeMode=single
  Divide : Product  Inputs=*/  OutDataTypeMode=single  OutScaling=2^-10
  Gain : Gain  Gain=-1
  delta : Outport
  wires:
  Gain/1 -> delta/1
  Add/1 -> Divide/1
  gamma/1 -> Add/2
  Constant5/1 -> Add/1
  Divide/1 -> Gain/1
  Constant1/1 -> Divide/2

== system SLUGS_Library/InnerLoop/Navigation/Compute WP Index/Compute Modified L1/Get Circles/compute delta Right Turn ==
  gamma : Inport
  Enable : EnablePort
  Add : Sum  Inputs=-+  OutDataTypeMode=single  OutScaling=2^-10
  Constant1 : Constant  Value=2  OutDataTypeMode=single
  Constant5 : Constant  Value=pi  OutDataTypeMode=single
  Divide : Product  Inputs=*/  OutDataTypeMode=single  OutScaling=2^-10
  delta : Outport
  wires:
  Divide/1 -> delta/1  "delta"
  gamma/1 -> Add/2
  Constant1/1 -> Divide/2
  Add/1 -> Divide/1
  Constant5/1 -> Add/1

== matlab function Singnal Routing & Conditioning/3D Filter/myMux Fun1 ==
  data: u1 input inherited; y output inherited; u2 input inherited; u3 input inherited
function y = myMux(u1, u2, u3)
% This block supports an embeddable subset of the MATLAB language.
% See the help menu for details. 

y = [u1(1); u2(1); u3(1)];

== matlab function Navigation/Compute Frenet/Select N Terms ==
  data: T input inherited; N output inherited
function N = getN(T)
% This block supports an embeddable subset of the MATLAB language.
% See the help menu for details. 

N = [-T(2); T(1); 0];

== matlab function Navigation/Compute WP Index/Compute Modified L1/Get Circles/Compute CCW Angle From 2 Vectors/Embedded MATLAB Function1 ==
  data: rawAngle input inherited; angle output inherited
function angle = mapToTwoPi(rawAngle)

 if(rawAngle < 0)
  angle = rawAngle + 2*pi;
 else
  angle = rawAngle;   
 end

== matlab function Compute CCW Angle From 2 Vectors/Embedded MATLAB Function1 ==
  data: rawAngle input inherited; angle output inherited
function angle = mapToTwoPi(rawAngle)

angle = rawAngle;

 if(angle < 0)
     while (angle <0)
        angle = angle + 2*pi;
     end;
 else
     while (angle > 2*pi)
        angle = angle - 2*pi;
     end
 end

== matlab function Subsystem3/Embedded MATLAB Function ==
  data: x input inherited; y input inherited; xDoty output inherited
function xDoty = myDot(x,y)
% This block supports an embeddable subset of the MATLAB language.
% See the help menu for details. 

xDoty = x(1)*y(1) + x(2)*y(2) + x(3)*y(3);

== matlab function Embedded MATLAB Function ==
  data: T1 input inherited; gamma output inherited; T2 input inherited
function gamma = computeAngle(T1, T2)
% This block supports an embeddable subset of the MATLAB language.
% See the help menu for details. 

gamma = (atan2(T1(2), T1(1)) - atan2(T2(2), T2(1)));

 if(gamma < 0)
  gamma = gamma + 2*pi;
 end

== matlab function Navigation/Compute WP Index/Embedded MATLAB Function ==
  data: wpStart input inherited; wpCount input inherited; wp0 output inherited; swIncrement input inherited; wp1 output inherited; wp2 output inherited; wpEnabl input inherited
function [wp0,wp1, wp2] = getNextWP(wpStart, wpCount, swIncrement, wpEnabl)

% Declare static variables
persistent fromWP;
persistent toWP;
persistent totoWP;

%initialize the static variables
if isempty(fromWP)
    fromWP = wpStart;
    toWP = fromWP+1;
    % check if there are more than 2 WPs
    if wpCount > toWP + 1
        totoWP = toWP+1;
    else
        totoWP = fromWP;
    end
end

%if WP Nav was just enabled
if wpEnabl == 1
    fromWP =0;
    toWP =1;
    totoWP = 2;
end;

% if there is a change of wp
if swIncrement == 1
    fromWP = toWP;
    toWP = totoWP;
    totoWP = totoWP +1;
    if (totoWP>wpCount)
        totoWP = wpStart;
    end
end

wp0 = fromWP;
wp1 = toWP;
wp2 = totoWP;

== matlab function InnerLoop/Navigation/Compute WP Index/Compute Modified L1/Get Circles/Compute Circles ==
  data: sd input inherited; O output inherited; cd input inherited; WP1 input inherited; R input inherited; T1 input inherited; P output inherited; Pch output inherited; T2 input inherited; PchB output inherited
function [O,P,Pch, PchB] = getO(sd, cd, WP1, R, T1, T2)
    % This block supports an embeddable subset of the MATLAB language.
    % See the help menu for details.

    % rotate the vector delta degrees
    r_vec = zeros(3,1);
    r_vec(1) = -T1(1)*cd -T1(2)*sd;
    r_vec(2) = T1(1)*sd -T1(2)*cd;

    %compute M
    if localAbs(sd)>0.01
        M = localAbs(R/sd);
    else
        M = single(0);
    end

    %find the distance from WP
    P = M*cd;

    % find the center of the circle
    O = WP1 + r_vec.*M;

    % find the tangent points
    Pch = WP1-T1*P;
    PchB = WP1 + T2*P;
end

function absVal = localAbs(x)
    if x < 0
        absVal = single(-1*x);
    else
        absVal = single(x);
    end
end

== matlab function InnerLoop/Navigation/Compute WP Index/Compute Modified L1/Get Circles/Compute CCW Angle From 2 Vectors/Embedded MATLAB Function1 ==
  data: rawAngle input inherited; angle output inherited
function angle = mapToTwoPi(rawAngle)

 if(rawAngle < 0)
  angle = rawAngle + 2*pi;
 else
  angle = rawAngle;   
 end

== matlab function InnerLoop/Navigation/Compute WP Index/Embedded MATLAB Function ==
  data: wpStart input inherited; wpCount input inherited; wp0 output inherited; swIncrement input inherited; wp1 output inherited; wp2 output inherited; wpEnabl input inherited
function [wp0,wp1, wp2] = getNextWP(wpStart, wpCount, swIncrement, wpEnabl)

% Declare static variables
persistent fromWP;
persistent toWP;
persistent totoWP;

%initialize the static variables
if isempty(fromWP)
    fromWP = uint8(wpStart);
    toWP = uint8(fromWP+1);
    % check if there are more than 2 WPs
    if wpCount > toWP + 1
        totoWP = uint8(toWP+1);
    else
        totoWP = uint8(fromWP);
    end
end

%if WP Nav was just enabled
if wpEnabl == 1
    fromWP = uint8(0);
    toWP = uint8(1);
    totoWP = uint8(2);
end;

% if there is a change of wp
if swIncrement == 1
    fromWP = toWP;
    toWP = totoWP;
    totoWP = totoWP +1;
    if (totoWP>wpCount)
        totoWP = wpStart;
    end
end

wp0 = fromWP;
wp1 = toWP;
wp2 = totoWP;

== matlab function negprotect ==
  data: val input inherited; zpVal output inherited
function zpVal = negProt(val)
% This block supports an embeddable subset of the MATLAB language.
% See the help menu for details. 

if val >= single(0.001)
    zpVal = val;
else
    zpVal = single(0.001);
end

== matlab function Navigation/Compute WP Index/Compute Modified L1/Get Circles/Compute Circles ==
  data: sd input inherited; O output inherited; cd input inherited; WP1 input inherited; R input inherited; T1 input inherited; P output inherited; Pch output inherited; T2 input inherited; PchB output inherited
function [O,P,Pch, PchB] = getO(sd, cd, WP1, R, T1, T2)
    % This block supports an embeddable subset of the MATLAB language.
    % See the help menu for details.

    % rotate the vector delta degrees
    r_vec = zeros(3,1);
    r_vec(1) = -T1(1)*cd -T1(2)*sd;
    r_vec(2) = T1(1)*sd -T1(2)*cd;

    %compute M
    if localAbs(sd)>0.01
        M = localAbs(R/sd);
    else
        M = 0;
    end

    %find the distance from WP
    P = M*cd;

    % find the center of the circle
    O = WP1 + r_vec.*M;

    % find the tangent points
    Pch = WP1-T1*P;
    PchB = WP1 + T2*P;
end

function absVal = localAbs(x)
    if x < 0
        absVal = -1*x;
    else
        absVal = x;
    end
end

== matlab function Subsystem1/negprotect ==
  data: val input inherited; zpVal output inherited
function zpVal = negProt(val)
% This block supports an embeddable subset of the MATLAB language.
% See the help menu for details. 

if val >= single(0.001)
    zpVal = val;
else
    zpVal = single(0.001);
end

== matlab function Navigation/Bank to Psi Dot/negprotect ==
  data: val input inherited; zpVal output inherited
function zpVal = negProt(val)
% This block supports an embeddable subset of the MATLAB language.
% See the help menu for details. 

if val >= single(0.001)
    zpVal = val;
else
    zpVal = single(0.001);
end

== matlab function Navigation/Park, Deyst & How Lat Accel Cmd/Compute Eta/negprotect ==
  data: val input inherited; zpVal output inherited
function zpVal = negProt(val)
% This block supports an embeddable subset of the MATLAB language.
% See the help menu for details. 

if val >= single(0.001)
    zpVal = val;
else
    zpVal = single(0.001);
end

== matlab function Navigation/Park, Deyst & How Lat Accel Cmd/Compute Eta/negprotect1 ==
  data: val input inherited; zpVal output inherited
function zpVal = negProt(val)
% This block supports an embeddable subset of the MATLAB language.
% See the help menu for details. 

if val >= single(0.001)
    zpVal = val;
else
    zpVal = single(0.001);
end

== matlab function Singnal Routing & Conditioning/myMux Fun3 ==
  data: u1 input inherited; y output inherited; u2 input inherited; u3 input inherited
function y = myMux(u1, u2, u3)
% This block supports an embeddable subset of the MATLAB language.
% See the help menu for details. 

y = [u1(1); u2(1); u3(1)];

== matlab function Singnal Routing & Conditioning/3D LowPass w/Initial Condition/myMux Fun1 ==
  data: u1 input inherited; y output inherited; u2 input inherited; u3 input inherited
function y = myMux(u1, u2, u3)
% This block supports an embeddable subset of the MATLAB language.
% See the help menu for details. 

y = [u1(1); u2(1); u3(1)];
